simulink model "ZT_VehCtrl_18B"  (R2018b)
settings: Solver=FixedStepAuto  StartTime=0.0  StopTime=inf  FixedStep=0.005  RelTol=1e-3
InitFcn:
  | mbd_mpc_consistency_checks(bdroot(gcs));
undefined symbols (not defined in the file): ANG_DEAD, BMS_NormalPwr, BrkPrsByBrkPct_TB_X, BrkPrsByBrkPct_TB_Y, DELAY_DISCHARGE, DELAY_RCUOFF, DRV_BACKWARD, DRV_BRAKE, DRV_FORWARD, DRV_NEUTRAL, DRV_PARK, DRV_UNPARK, DRV_ZEROTURN, EPB_LOCK, EPB_UNLOCK, ExtraLoadPwr, FanOff, fifo_0_vect, fifo_1_vect, HiFanReq, HV_finished, HV_No_Active, HV_POWER_OFF, HV_POWER_ON, HVDown, HVON, KaTLS_v_DrgUp_X_VehSpd, KeFTM_s_Way1OffDlyTime, KeFTM_TK_Way1CoolLv2OffBatTemp, KeFTM_TK_Way1CoolLv2OffMtrTemp, KeFTM_TK_Way1CoolLv2OnBatTemp, KeFTM_TK_Way1CoolLv2OnMtrTemp, KeFTM_TK_Way1CoolLv3OffBatTemp, KeFTM_TK_Way1CoolLv3OffMtrTemp, KeFTM_TK_Way1CoolLv3OnBatTemp, KeFTM_TK_Way1CoolLv3OnMtrTemp, KeFTM_TK_Way1CoolLv4OffBatTemp, KeFTM_TK_Way1CoolLv4OffMtrTemp, KeFTM_TK_Way1CoolLv4OnBatTemp, KeFTM_TK_Way1CoolLv4OnMtrTemp, Kp1, Kp2, LowFanReq, LQFP, MtrPwrFactor_RCU, MtrPwrHighToMidThd, MtrPwrLowToMidThd, MtrPwrMidToHighThd, MtrPwrMidToLowThd, MtrTrqMax, PCT_DEAD, Precharge, PTO_1000, PTO_540, pts1_fifo_0_vect, pts1_fifo_1_vect, pts2_fifo_0_vect, pts2_fifo_1_vect, pts3_fifo_0_vect, pts3_fifo_1_vect ... (+24)
libraries: mbd_mpc574x_ec_toolbox x124, canmsglib x72, simulink x57
(part 10 of 11)

== system ZT_VehCtrl_18B/SigOut/GPIO /PWM_OUT/PWM Configuration and Frequency Update4 ==
  PWM A : Inport
  Fre : Inport  Port=2
  Add : Sum  Inputs=+-
  Constant : Constant
  Constant1 : Constant  Commented=on  Value=200
  Data Type Conversion : DataTypeConversion
  Data Type Conversion1 : DataTypeConversion  Commented=on
  FlexPWM_Config : mbd_mpc574x_ec_toolbox/Motor Control Blocks/FlexPWM Blocks/FlexPWM_Config  Priority=1  pwmModule=0  pwmSubmodule=1  pwmMode=Center aligned PWM  pwmPair=Independent  pwmCompSource=PWM23  pwmCounterInit=Local sync (PWMX)  pwmClockSource=Peripheral clock  pwmUnits=Hz  pwmFrequency=200  pwmPeriod=25000  pwmPrescaler=Divide by 16  pwmDtUnits=Nanoseconds  pwmDtNs=50  pwmDtTicks=4  pwmReloadLogic=Full Cycle  pwmReloadFrequency=Every 1 PWM opportunity  pwmTriggeringSignal=Local force signal  pwmDutyCycleOutSim=off  pwmStartAfterInit=on  pwmShowAdvOpts=off  pwmPinA=PTC7: [PWM0_A1 | FlexPWM_0 Channel A Input/Output 1]  pwmPinB=None  pwmPolarityA=off  pwmPolarityB=off  pwmAInitialVal=0.25  pwmBInitialVal=0.25  pwmAShift=0  pwmBShift=0  trgReloadISR=off  trgVal0=off  trgVal1=off  trgVal2=off  trgVal3=off  trgVal4=off  trgVal5=off  trgReloadErrorISR=off  pwmPinFault=None  PwmFaultEnISR=off  pwmFaultEnA=off  pwmFaultEnB=off
  FlexPWM_Frequency_Update : mbd_mpc574x_ec_toolbox/Motor Control Blocks/FlexPWM Blocks/FlexPWM_Frequency_Update  Priority=1  Commented=on  pwmModule=0  pwmSubmodule0=off  pwmSubmodule1=on  pwmSubmodule2=off  pwmSubmodule3=off  pwmUnits=Hz
  Terminator : Terminator
  wires:
  PWM A/1 -> Add/2
  Add/1 -> Data Type Conversion/1
  Constant/1 -> Add/1
  Data Type Conversion/1 -> FlexPWM_Config/1
  Fre/1 -> Terminator/1
  Constant1/1 -> Data Type Conversion1/1
  Data Type Conversion1/1 -> FlexPWM_Frequency_Update/1

== system ZT_VehCtrl_18B/SigOut/GPIO /SPI0: LS09_14_15_16_1_2_11_4/LS_CTRL ==
  Enable : EnablePort
  Data Type Conversion3 : DataTypeConversion
  Data Type Conversion4 : DataTypeConversion
  Demux1 : Demux  Outputs=2
  If Action Subsystem1 : Subsystem  TreatAsAtomicUnit=on
  SPI_Master_Transfer_To1 : mbd_mpc574x_ec_toolbox/Communication Blocks/SPI Blocks/SPI_Master_Transfer  Priority=2  InstanceNumber=0  xfermode=Non blocking  timeout=50  spi_upd=on  WhichPCS=5
  Terminator : Terminator
  Terminator1 : Terminator
  Vector Concatenate1 : Concatenate
  wires:
  Vector Concatenate1/1 -> SPI_Master_Transfer_To1/1
  SPI_Master_Transfer_To1/1 -> Demux1/1
  Demux1/2 -> Data Type Conversion4/1
  Data Type Conversion3/1 -> Terminator/1
  Data Type Conversion4/1 -> Terminator1/1
  Demux1/1 -> Data Type Conversion3/1
  If Action Subsystem1/1(Out1) -> Vector Concatenate1/1
  If Action Subsystem1/2(Out2) -> Vector Concatenate1/2

== system ZT_VehCtrl_18B/SigOut/GPIO /SPI0: LS09_14_15_16_1_2_11_4/LS_CTRL1 ==
  Enable : EnablePort
  Data Type Conversion3 : DataTypeConversion
  Data Type Conversion4 : DataTypeConversion
  Demux1 : Demux  Outputs=2
  If Action Subsystem1 : Subsystem  TreatAsAtomicUnit=on
  SPI_Master_Transfer_To1 : mbd_mpc574x_ec_toolbox/Communication Blocks/SPI Blocks/SPI_Master_Transfer  Priority=2  InstanceNumber=0  xfermode=Non blocking  timeout=50  spi_upd=on  WhichPCS=1
  Terminator : Terminator
  Terminator1 : Terminator
  Vector Concatenate1 : Concatenate
  wires:
  Demux1/1 -> Data Type Conversion3/1
  Data Type Conversion4/1 -> Terminator1/1
  Data Type Conversion3/1 -> Terminator/1
  Demux1/2 -> Data Type Conversion4/1
  SPI_Master_Transfer_To1/1 -> Demux1/1
  Vector Concatenate1/1 -> SPI_Master_Transfer_To1/1
  If Action Subsystem1/2(Out2) -> Vector Concatenate1/2
  If Action Subsystem1/1(Out1) -> Vector Concatenate1/1

== system ZT_VehCtrl_18B/SigOut/GPIO /SPI3: LS03_06_07_08_10_12_13_17_18_19/Subsystem ==
  Enable : EnablePort
  Data Type Conversion : DataTypeConversion  OutDataTypeStr=uint8
  Data Type Conversion1 : DataTypeConversion  OutDataTypeStr=uint8
  Demux2 : Demux  Outputs=2
  SPI_Master_Transfer_To2 : mbd_mpc574x_ec_toolbox/Communication Blocks/SPI Blocks/SPI_Master_Transfer  Priority=2  InstanceNumber=3  xfermode=Non blocking  timeout=50  spi_upd=on  WhichPCS=3
  Terminator2 : Terminator
  Terminator3 : Terminator
  Vector Concatenate2 : Concatenate
  控制 : Subsystem  TreatAsAtomicUnit=on
  wires:
  Data Type Conversion1/1 -> Terminator3/1
  控制/2(Out2) -> Vector Concatenate2/2
  Demux2/1 -> Data Type Conversion/1
  Vector Concatenate2/1 -> SPI_Master_Transfer_To2/1
  Demux2/2 -> Data Type Conversion1/1
  Data Type Conversion/1 -> Terminator2/1
  控制/1(Out1) -> Vector Concatenate2/1
  SPI_Master_Transfer_To2/1 -> Demux2/1

== system ZT_VehCtrl_18B/VehCtrl/MontionControl/DriveControl/Brake ==
  VehBrkTgt : Inport
  In2 : Inport  Port=2
  1-D Lookup Table : Lookup_n-D  NumberOfTableDimensions=1  BreakpointsForDimension1=BrkPrsByBrkPct_TB_X  Table=BrkPrsByBrkPct_TB_Y  InternalRulePriority=Speed  RndMeth=Simplest  InputSameDT=on
  Bus Selector : BusSelector  OutputSignals=NonDrive
  Constant : Constant
  Gain : Gain  Gain=0.01
  Switch : Switch  Criteria=u2 > Threshold
  BrkPrsTgt : Outport
  wires:
  VehBrkTgt/1 -> Gain/1  "VehBrkTgt"
  1-D Lookup Table/1 -> BrkPrsTgt/1
  Gain/1 -> Switch/3
  Switch/1 -> 1-D Lookup Table/1
  In2/1 -> Bus Selector/1
  Bus Selector/1 -> Switch/2  "<NonDrive>"
  Constant/1 -> Switch/1

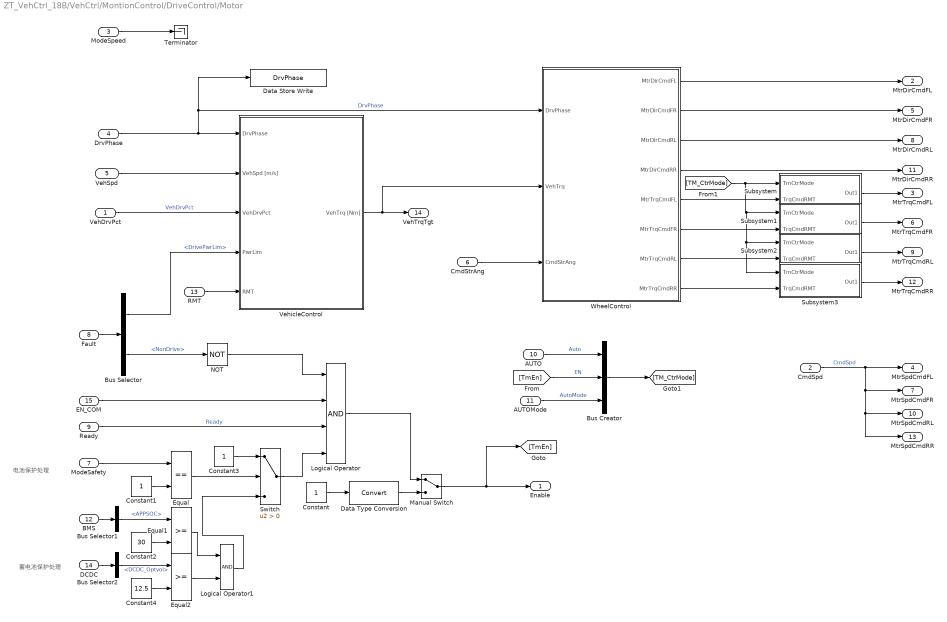
== system ZT_VehCtrl_18B/VehCtrl/MontionControl/DriveControl/Motor ==
  note: 电池保护处理
  note: 蓄电池保护处理
  VehDrvPct : Inport
  CmdSpd : Inport  Port=2
  ModeSpeed : Inport  Port=3
  DrvPhase : Inport  Port=4
  VehSpd : Inport  Port=5
  CmdStrAng : Inport  Port=6
  ModeSafety : Inport  Port=7
  Fault : Inport  Port=8
  Ready : Inport  Port=9
  AUTO : Inport  Port=10
  AUTOMode : Inport  Port=11
  BMS : Inport  Port=12
  RMT : Inport  Port=13
  DCDC : Inport  Port=14
  EN_COM : Inport  Port=15
  Bus Creator : BusCreator  Inputs=3
  Bus Selector : BusSelector  OutputSignals=DrivePwrLim,NonDrive
  Bus Selector1 : BusSelector  OutputSignals=BMS Power Infor.APPSOC
  Bus Selector2 : BusSelector  OutputSignals=DCDC_Optvol
  Constant : Constant
  Constant1 : Constant  OutDataTypeStr=boolean
  Constant2 : Constant  Value=30  OutDataTypeStr=boolean
  Constant3 : Constant  OutDataTypeStr=boolean
  Constant4 : Constant  Value=12.5  OutDataTypeStr=boolean
  Data Store Write : DataStoreWrite  DataStoreName=DrvPhase
  Data Type Conversion : DataTypeConversion
  Equal : RelationalOperator  Operator===  OutDataTypeStr=boolean  RndMeth=Simplest
  Equal1 : RelationalOperator  OutDataTypeStr=boolean  RndMeth=Simplest
  Equal2 : RelationalOperator  OutDataTypeStr=boolean  RndMeth=Simplest
  Logical Operator : Logic  Inputs=4  AllPortsSameDT=off  OutDataTypeStr=boolean
  Logical Operator1 : Logic  AllPortsSameDT=off  OutDataTypeStr=boolean
  Manual Switch : ManualSwitch
  NOT : Logic  Operator=NOT  IconShape=distinctive  AllPortsSameDT=off  OutDataTypeStr=boolean
  Subsystem : Subsystem
  Subsystem1 : Subsystem
  Subsystem2 : Subsystem
  Subsystem3 : Subsystem
  Switch : Switch  Criteria=u2 > Threshold
  Terminator : Terminator
  VehicleControl : Subsystem  TreatAsAtomicUnit=on
  WheelControl : Subsystem
  Enable : Outport
  MtrDirCmdFL : Outport  Port=2
  MtrTrqCmdFL : Outport  Port=3
  MtrSpdCmdFL : Outport  Port=4
  MtrDirCmdFR : Outport  Port=5
  MtrTrqCmdFR : Outport  Port=6
  MtrSpdCmdFR : Outport  Port=7
  MtrDirCmdRL : Outport  Port=8
  MtrTrqCmdRL : Outport  Port=9
  MtrSpdCmdRL : Outport  Port=10
  MtrDirCmdRR : Outport  Port=11
  MtrTrqCmdRR : Outport  Port=12
  MtrSpdCmdRR : Outport  Port=13
  VehTrqTgt : Outport  Port=14
  wires:
  VehSpd/1 -> VehicleControl/2(VehSpd [m/s])
  VehDrvPct/1 -> VehicleControl/3(VehDrvPct)  "VehDrvPct"
  DrvPhase/1 -> Data Store Write/1, WheelControl/1(DrvPhase), VehicleControl/1(DrvPhase)  "DrvPhase"
  CmdSpd/1 -> MtrSpdCmdRR/1, MtrSpdCmdRL/1, MtrSpdCmdFR/1, MtrSpdCmdFL/1  "CmdSpd"
  WheelControl/1(MtrDirCmdFL) -> MtrDirCmdFL/1
  WheelControl/2(MtrDirCmdFR) -> MtrDirCmdFR/1
  WheelControl/3(MtrDirCmdRL) -> MtrDirCmdRL/1
  WheelControl/4(MtrDirCmdRR) -> MtrDirCmdRR/1
  Fault/1 -> Bus Selector/1
  Bus Selector/1 -> VehicleControl/4(PwrLim)  "<DrivePwrLim>"
  Bus Selector/2 -> NOT/1  "<NonDrive>"
  NOT/1 -> Logical Operator/1
  Ready/1 -> Logical Operator/3  "Ready"
  Manual Switch/1 -> [TmEn], Enable/1
  VehicleControl/1(VehTrq [Nm]) -> WheelControl/2(VehTrq), VehTrqTgt/1
  CmdStrAng/1 -> WheelControl/3(CmdStrAng)
  WheelControl/5(MtrTrqCmdFL) -> Subsystem/2(TrqCmdRMT)
  WheelControl/6(MtrTrqCmdFR) -> Subsystem1/2(TrqCmdRMT)
  WheelControl/7(MtrTrqCmdRL) -> Subsystem2/2(TrqCmdRMT)
  WheelControl/8(MtrTrqCmdRR) -> Subsystem3/2(TrqCmdRMT)
  ModeSpeed/1 -> Terminator/1
  ModeSafety/1 -> Equal/1
  Constant1/1 -> Equal/2
  Equal/1 -> Switch/2
  Constant2/1 -> Equal1/2
  Logical Operator1/1 -> Switch/3
  Constant3/1 -> Switch/1
  Switch/1 -> Logical Operator/4
  AUTO/1 -> Bus Creator/1  "Auto"
  AUTOMode/1 -> Bus Creator/3  "AutoMode"
  BMS/1 -> Bus Selector1/1
  Bus Selector1/1 -> Equal1/1  "<APPSOC>"
  RMT/1 -> VehicleControl/5(RMT)
  Equal1/1 -> Logical Operator1/1
  Constant4/1 -> Equal2/2
  Equal2/1 -> Logical Operator1/2
  DCDC/1 -> Bus Selector2/1
  Bus Selector2/1 -> Equal2/1  "<DCDC_Optvol>"
  [TmEn] -> Bus Creator/2  "EN"
  Subsystem/1(Out1) -> MtrTrqCmdFL/1
  Bus Creator/1 -> [TM_CtrMode]
  [TM_CtrMode] -> Subsystem1/1(TmCtrMode), Subsystem3/1(TmCtrMode), Subsystem2/1(TmCtrMode), Subsystem/1(TmCtrMode)
  Subsystem1/1(Out1) -> MtrTrqCmdFR/1
  Subsystem2/1(Out1) -> MtrTrqCmdRL/1
  Subsystem3/1(Out1) -> MtrTrqCmdRR/1
  Constant/1 -> Data Type Conversion/1
  Data Type Conversion/1 -> Manual Switch/2
  Logical Operator/1 -> Manual Switch/1
  EN_COM/1 -> Logical Operator/2

== system ZT_VehCtrl_18B/VehCtrl/MontionControl/PtoControl/Subsystem ==
  ModeSpeed : Inport
  DirCmd : Inport  Port=2
  Add : Sum
  Constant : Constant  Value=16  OutDataTypeStr=uint8
  Constant1 : Constant  Value=4  OutDataTypeStr=uint8
  Constant2 : Constant  Value=32  OutDataTypeStr=uint8
  Constant3 : Constant  Value=0  OutDataTypeStr=uint8
  Switch : Switch  Criteria=u2 > Threshold
  Switch1 : Switch  Criteria=u2 > Threshold
  ModeReq : Outport
  wires:
  DirCmd/1 -> Switch/2
  Constant/1 -> Switch/1
  Constant1/1 -> Switch/3
  ModeSpeed/1 -> Switch1/2
  Constant2/1 -> Switch1/1
  Constant3/1 -> Switch1/3
  Switch1/1 -> Add/1
  Switch/1 -> Add/2
  Add/1 -> ModeReq/1

== system ZT_VehCtrl_18B/VehCtrl/MontionControl/PtoControl/Subsystem1 ==
  <RMT_PtoMode> : Inport
  Constant : Constant  Value=PTO_540
  Constant1 : Constant  Value=PTO_1000
  Constant2 : Constant  Value=540  OutDataTypeStr=single
  Constant3 : Constant  Value=1000  OutDataTypeStr=single
  Constant4 : Constant  Value=0  OutDataTypeStr=single
  Gain : Gain
  GreaterThan : RelationalOperator  Operator===  OutDataTypeStr=boolean  RndMeth=Simplest
  GreaterThan1 : RelationalOperator  Operator===  OutDataTypeStr=boolean  RndMeth=Simplest
  Switch : Switch  Criteria=u2 > Threshold
  Switch1 : Switch  Criteria=u2 > Threshold
  MtrSpdCmd : Outport
  wires:
  Switch1/1 -> Switch/3
  Constant4/1 -> Switch1/3
  Constant1/1 -> GreaterThan1/2
  GreaterThan1/1 -> Switch1/2
  Constant2/1 -> Switch/1
  Constant3/1 -> Switch1/1
  Constant/1 -> GreaterThan/2
  GreaterThan/1 -> Switch/2
  <RMT_PtoMode>/1 -> GreaterThan1/1, GreaterThan/1
  Switch/1 -> Gain/1
  Gain/1 -> MtrSpdCmd/1  "MtrSpdCmd"

== system ZT_VehCtrl_18B/VehCtrl/MontionControl/ValveControl/BrakeSys ==
  BrkPrsTgt : Inport
  BrkPrs : Inport  Port=2
  Chart : Stateflow chart  Commented=on  TreatAsAtomicUnit=on
  BrkValve : Outport
  wires:
  BrkPrs/1 -> Chart/1(BrkPrs)
  BrkPrsTgt/1 -> BrkValve/1, Chart/2(BrkPrsTgt)

== system ZT_VehCtrl_18B/VehCtrl/MontionControl/ValveControl/EpbSys ==
  EpbSt : Inport
  EpbValve : Outport
  wires:
  EpbSt/1 -> EpbValve/1

== system ZT_VehCtrl_18B/VehCtrl/MontionControl/ValveControl/PumpSys ==
  Ready : Inport
  Compare To Zero : simulink/Logic and Bit Operations/Compare To Zero  relop=>  OutDataTypeStr=boolean
  Pump : Outport
  wires:
  Compare To Zero/1 -> Pump/1
  Ready/1 -> Compare To Zero/1

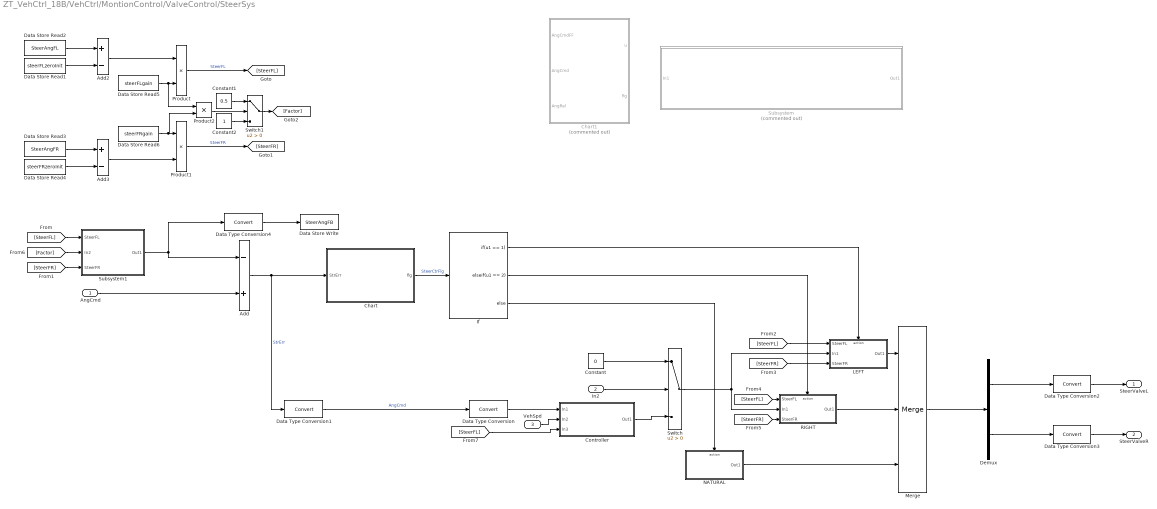
== system ZT_VehCtrl_18B/VehCtrl/MontionControl/ValveControl/SteerSys ==
  AngCmd : Inport
  In2 : Inport  Port=2
  VehSpd : Inport  Port=3
  Add : Sum  Inputs=-+
  Add2 : Sum  Inputs=+-
  Add3 : Sum  Inputs=+-
  Chart : Stateflow chart  TreatAsAtomicUnit=on
  Chart1 : Stateflow chart  Commented=on  TreatAsAtomicUnit=on
  Constant : Constant  Value=0  OutDataTypeStr=single
  Constant1 : Constant  Value=0.5  OutDataTypeStr=single
  Constant2 : Constant  OutDataTypeStr=single
  Controller : Subsystem
  Data Store Read1 : DataStoreRead  DataStoreName=steerFLzeroInit
  Data Store Read2 : DataStoreRead  DataStoreName=SteerAngFL
  Data Store Read3 : DataStoreRead  DataStoreName=SteerAngFR
  Data Store Read4 : DataStoreRead  DataStoreName=steerFRzeroInit
  Data Store Read5 : DataStoreRead  DataStoreName=steerFLgain
  Data Store Read6 : DataStoreRead  DataStoreName=steerFRgain
  Data Store Write : DataStoreWrite  DataStoreName=SteerAngFB
  Data Type Conversion{,1..4} (5 alike) : DataTypeConversion
  Demux : Demux  Outputs=2
  If : If  IfExpression=u1 == 1  ElseIfExpressions=u1 == 2
  LEFT : Subsystem  TreatAsAtomicUnit=on
  Merge : Merge  Inputs=3
  "NATURAL " : Subsystem  TreatAsAtomicUnit=on
  Product : Product
  Product1 : Product
  Product2 : Product
  RIGHT : Subsystem  TreatAsAtomicUnit=on
  Subsystem : Subsystem  Commented=on
  Subsystem1 : Subsystem
  Switch : Switch  Criteria=u2 > Threshold
  Switch1 : Switch  Criteria=u2 > Threshold
  SteerValveL : Outport
  SteerValveR : Outport  Port=2
  wires:
  If/1 -> LEFT/Action
  Switch/1 -> LEFT/2(In1), RIGHT/2(In1)
  If/2 -> RIGHT/Action
  If/3 -> "NATURAL "/Action
  RIGHT/1(Out1) -> Merge/2
  "NATURAL "/1(Out1) -> Merge/3
  LEFT/1(Out1) -> Merge/1
  Merge/1 -> Demux/1
  Data Type Conversion2/1 -> SteerValveL/1
  Data Type Conversion3/1 -> SteerValveR/1
  Demux/1 -> Data Type Conversion2/1
  Demux/2 -> Data Type Conversion3/1
  Subsystem1/1(Out1) -> Add/1, Data Type Conversion4/1
  Data Type Conversion4/1 -> Data Store Write/1
  Add/1 -> Chart/1(StrErr), Data Type Conversion1/1  "StrErr"
  Chart/1(flg) -> If/1  "SteerCtrFlg"
  Controller/1(Out1) -> Switch/3
  In2/1 -> Switch/2
  Constant/1 -> Switch/1
  AngCmd/1 -> Add/2
  VehSpd/1 -> Controller/2(In2)
  Data Type Conversion1/1 -> Data Type Conversion/1  "AngCmd"
  Add3/1 -> Product1/2
  Data Store Read4/1 -> Add3/2
  Data Store Read5/1 -> Product2/1, Product/2
  Data Store Read2/1 -> Add2/1
  Add2/1 -> Product/1
  Product1/1 -> [SteerFR]  "SteerFR"
  Data Store Read6/1 -> Product2/2, Product1/1
  Data Store Read1/1 -> Add2/2
  Data Store Read3/1 -> Add3/1
  Product/1 -> [SteerFL]  "SteerFL"
  [SteerFL] -> Subsystem1/1(SteerFL)
  [SteerFR] -> Subsystem1/3("SteerFR ")
  [SteerFR] -> LEFT/3(SteerFR)
  [SteerFL] -> LEFT/1("SteerFL ")
  [SteerFL] -> RIGHT/1(SteerFL)
  [SteerFR] -> RIGHT/3(SteerFR)
  Product2/1 -> Switch1/2
  Constant1/1 -> Switch1/1
  Constant2/1 -> Switch1/3
  Switch1/1 -> [Factor]
  [Factor] -> Subsystem1/2(In2)
  Data Type Conversion/1 -> Controller/1(In1)
  [SteerFL] -> Controller/3(In3)

== system ZT_VehCtrl_18B/VehCtrl/MontionControl/ValveControl/SuspesionSys ==
  note: 由于没有高度或长度传感器，初期为开环控制；
      | 后续考虑是否可以增加传感器，构建闭环控制。
  SuspSt : Inport
  ModeSafety : Inport  Port=2
  Constant{,1,3..4} (4 alike) : Constant  Value=false  OutDataTypeStr=boolean
  Constant2 : Constant  Value=true  OutDataTypeStr=boolean
  Constant5 : Constant  Value=true  OutDataTypeStr=boolean
  Constant6 : Constant  Value=0
  Data Type Conversion : DataTypeConversion
  Data Type Conversion1 : DataTypeConversion
  Data Type Conversion2 : DataTypeConversion  OutDataTypeStr=uint8
  Data Type Conversion3 : DataTypeConversion  OutDataTypeStr=uint8
  Data Type Conversion4 : DataTypeConversion  OutDataTypeStr=uint8
  Demux : Demux  Outputs=2
  Multiport Switch : MultiPortSwitch  DataPortOrder=Zero-based contiguous  zeroidx=on
  Mux : Mux  Inputs=2
  Mux1 : Mux  Inputs=2
  Mux2 : Mux  Inputs=2
  Switch1 : Switch  Criteria=u2 > Threshold
  SuspUpValve : Outport
  SuspDownValve : Outport  Port=2
  wires:
  Mux/1 -> Multiport Switch/2
  Mux1/1 -> Multiport Switch/3
  Mux2/1 -> Multiport Switch/4
  Constant/1 -> Mux/1
  Constant1/1 -> Mux/2
  Constant3/1 -> Mux1/2
  Constant2/1 -> Mux1/1
  Constant4/1 -> Mux2/1
  Constant5/1 -> Mux2/2
  Switch1/1 -> Data Type Conversion4/1
  Multiport Switch/1 -> Demux/1
  Demux/2 -> Data Type Conversion1/1
  Demux/1 -> Data Type Conversion/1
  Data Type Conversion/1 -> SuspUpValve/1
  Data Type Conversion1/1 -> SuspDownValve/1
  Data Type Conversion4/1 -> Multiport Switch/1  "suspmodeCtrl"
  ModeSafety/1 -> Switch1/2
  SuspSt/1 -> Data Type Conversion2/1
  Data Type Conversion2/1 -> Switch1/1
  Data Type Conversion3/1 -> Switch1/3
  Constant6/1 -> Data Type Conversion3/1

== system ZT_VehCtrl_18B/VehCtrl/MontionControl/ValveControl/WidthSys ==
  ModeSafety : Inport
  <RMT_ModeWidth> : Inport  Port=2
  Constant{,1,3..4} (4 alike) : Constant  Value=false  OutDataTypeStr=boolean
  Constant2 : Constant  Value=true  OutDataTypeStr=boolean
  Constant5 : Constant  Value=true  OutDataTypeStr=boolean
  Constant6 : Constant  Value=0  OutDataTypeStr=boolean
  Data Type Conversion : DataTypeConversion
  Data Type Conversion1 : DataTypeConversion
  Data Type Conversion2 : DataTypeConversion  OutDataTypeStr=uint8
  Data Type Conversion3 : DataTypeConversion  OutDataTypeStr=uint8
  Data Type Conversion4 : DataTypeConversion  OutDataTypeStr=uint8
  Demux : Demux  Outputs=2
  Multiport Switch : MultiPortSwitch  DataPortOrder=Zero-based contiguous  zeroidx=on
  Mux : Mux  Inputs=2
  Mux1 : Mux  Inputs=2
  Mux2 : Mux  Inputs=2
  Switch1 : Switch  Criteria=u2 > Threshold
  WidthLengthenValve : Outport
  WidthShortenValve : Outport  Port=2
  wires:
  Multiport Switch/1 -> Demux/1
  Demux/1 -> Data Type Conversion/1
  Demux/2 -> Data Type Conversion1/1
  Constant/1 -> Mux/1
  Mux2/1 -> Multiport Switch/4
  Constant2/1 -> Mux1/1
  Constant3/1 -> Mux1/2
  Mux1/1 -> Multiport Switch/3
  Mux/1 -> Multiport Switch/2
  Constant1/1 -> Mux/2
  Constant5/1 -> Mux2/2
  Constant4/1 -> Mux2/1
  Data Type Conversion/1 -> WidthLengthenValve/1
  Data Type Conversion1/1 -> WidthShortenValve/1
  ModeSafety/1 -> Switch1/2
  <RMT_ModeWidth>/1 -> Data Type Conversion2/1
  Constant6/1 -> Data Type Conversion3/1
  Switch1/1 -> Data Type Conversion4/1
  Data Type Conversion2/1 -> Switch1/1
  Data Type Conversion3/1 -> Switch1/3
  Data Type Conversion4/1 -> Multiport Switch/1  "widthmodeCtrl"

== system ZT_VehCtrl_18B/VehCtrl/TempertureControl/ThermFR_RRvRead1/Cnt_To_s ==
  In1 : Inport
  Constant1 : Constant  Value=200  OutDataTypeStr=uint8
  Data Type Conversion2 : DataTypeConversion  OutDataTypeStr=uint32
  Product1 : Product  OutDataTypeStr=fixdt(0,16,0.1,0)  RndMeth=Zero
  Out1 : Outport
  wires:
  Data Type Conversion2/1 -> Out1/1
  In1/1 -> Product1/1
  Product1/1 -> Data Type Conversion2/1
  Constant1/1 -> Product1/2

== system ZT_VehCtrl_18B/VehCtrl/TempertureControl/ThermFR_RRvRead2/Cnt_To_s ==
  In1 : Inport
  Constant1 : Constant  Value=200  OutDataTypeStr=uint8
  Data Type Conversion2 : DataTypeConversion  OutDataTypeStr=uint32
  Product1 : Product  OutDataTypeStr=fixdt(0,16,0.1,0)  RndMeth=Zero
  Out1 : Outport
  wires:
  Constant1/1 -> Product1/2
  Product1/1 -> Data Type Conversion2/1
  In1/1 -> Product1/1
  Data Type Conversion2/1 -> Out1/1

== system ZT_VehCtrl_18B/VehCtrl/TempertureControl/ThermLvRead3/Cnt_To_s ==
  In1 : Inport
  Constant1 : Constant  Value=200  OutDataTypeStr=uint8
  Data Type Conversion2 : DataTypeConversion  OutDataTypeStr=uint32
  Product1 : Product  OutDataTypeStr=fixdt(0,16,0.1,0)  RndMeth=Zero
  Out1 : Outport
  wires:
  Constant1/1 -> Product1/2
  Product1/1 -> Data Type Conversion2/1
  In1/1 -> Product1/1
  Data Type Conversion2/1 -> Out1/1

== system ZT_VehCtrl_18B/SigIn/PWM/Subsystem/eTimer Configuration and Signal Measurements/Subsystem_capture ==
  In1 : Inport
  function : TriggerPort  TriggerType=function-call  VariantControl=Variant
  Terminator : Terminator
  eTimer_Arm_Capture : mbd_mpc574x_ec_toolbox/Motor Control Blocks/eTIMER Blocks/eTimer_Arm_Capture  etimerModule=0  etimerChannel=1  etimerArmAction=Stop
  eTimer_Capture : mbd_mpc574x_ec_toolbox/Motor Control Blocks/eTIMER Blocks/eTimer_Capture  etimerModule=0  etimerChannel=1
  Out1 : Outport  OutDataTypeStr=uint16
  Out2 : Outport  Port=2  OutDataTypeStr=uint16
  Out3 : Outport  Port=3  OutDataTypeStr=uint16
  Out4 : Outport  Port=4  OutDataTypeStr=uint16
  wires:
  eTimer_Capture/1 -> Out1/1
  eTimer_Capture/4 -> Out4/1
  eTimer_Capture/3 -> Out3/1
  eTimer_Capture/2 -> Out2/1
  In1/1 -> Terminator/1

== system ZT_VehCtrl_18B/SigOut/GPIO /SPI0: LS09_14_15_16_1_2_11_4/LS_CTRL/If Action Subsystem1 ==
  Add : Sum  Inputs=++++
  Constant1 : Constant  Value=128  OutDataTypeStr=uint8
  Constant2 : Constant  Value=64  OutDataTypeStr=uint8
  Constant3 : Constant  Value=32  OutDataTypeStr=uint8
  Constant4 : Constant  Value=16  OutDataTypeStr=uint8
  Constant5 : Constant  Value=8  OutDataTypeStr=uint8
  Constant6 : Constant  Value=4  OutDataTypeStr=uint8
  Constant7 : Constant  Value=2  OutDataTypeStr=uint8
  Constant8 : Constant  OutDataTypeStr=uint8
  Constant9 : Constant  Value=128  OutDataTypeStr=uint8
  Data Store Read : DataStoreRead  DataStoreName=LS004
  Data Store Read4 : DataStoreRead  DataStoreName=LS011
  Data Store Read5 : DataStoreRead  DataStoreName=LS001
  Data Store Read6 : DataStoreRead  DataStoreName=LS002
  Data Type Conversion : DataTypeConversion
  Data Type Conversion1 : DataTypeConversion
  Switch{,1..3} (4 alike) : Switch  Criteria=u2 > Threshold
  Out1 : Outport
  Out2 : Outport  Port=2
  wires:
  Constant2/1 -> Switch/3
  Constant1/1 -> Switch/1
  Add/1 -> Data Type Conversion1/1
  Data Store Read6/1 -> Switch/2
  Constant7/1 -> Switch3/1
  Switch1/1 -> Add/2
  Constant5/1 -> Switch2/1
  Switch/1 -> Add/1
  Constant4/1 -> Switch1/3
  Data Store Read/1 -> Switch3/2
  Switch2/1 -> Add/3
  Data Store Read4/1 -> Switch2/2
  Switch3/1 -> Add/4
  Constant3/1 -> Switch1/1
  Data Store Read5/1 -> Switch1/2
  Constant8/1 -> Switch3/3
  Constant9/1 -> Data Type Conversion/1
  Constant6/1 -> Switch2/3
  Data Type Conversion/1 -> Out1/1
  Data Type Conversion1/1 -> Out2/1

== system ZT_VehCtrl_18B/SigOut/GPIO /SPI0: LS09_14_15_16_1_2_11_4/LS_CTRL1/If Action Subsystem1 ==
  Add : Sum  Inputs=++++
  Constant1 : Constant  Value=128  OutDataTypeStr=uint8
  Constant2 : Constant  Value=64  OutDataTypeStr=uint8
  Constant3 : Constant  Value=32  OutDataTypeStr=uint8
  Constant4 : Constant  Value=16  OutDataTypeStr=uint8
  Constant5 : Constant  Value=8  OutDataTypeStr=uint8
  Constant6 : Constant  Value=4  OutDataTypeStr=uint8
  Constant7 : Constant  Value=2  OutDataTypeStr=uint8
  Constant8 : Constant  OutDataTypeStr=uint8
  Constant9 : Constant  Value=128  OutDataTypeStr=uint8
  Data Store Read : DataStoreRead  DataStoreName=LS014
  Data Store Read4 : DataStoreRead  DataStoreName=LS015
  Data Store Read5 : DataStoreRead  DataStoreName=LS009
  Data Store Read6 : DataStoreRead  DataStoreName=LS016
  Data Type Conversion : DataTypeConversion
  Data Type Conversion1 : DataTypeConversion
  Switch{,1..3} (4 alike) : Switch  Criteria=u2 > Threshold
  Out1 : Outport
  Out2 : Outport  Port=2
  wires:
  Data Type Conversion1/1 -> Out2/1
  Data Type Conversion/1 -> Out1/1
  Constant6/1 -> Switch2/3
  Constant9/1 -> Data Type Conversion/1
  Constant8/1 -> Switch3/3
  Data Store Read5/1 -> Switch1/2
  Constant3/1 -> Switch1/1
  Switch3/1 -> Add/4
  Data Store Read4/1 -> Switch2/2
  Switch2/1 -> Add/3
  Data Store Read/1 -> Switch3/2
  Constant4/1 -> Switch1/3
  Switch/1 -> Add/1
  Constant5/1 -> Switch2/1
  Switch1/1 -> Add/2
  Constant7/1 -> Switch3/1
  Data Store Read6/1 -> Switch/2
  Add/1 -> Data Type Conversion1/1
  Constant1/1 -> Switch/1
  Constant2/1 -> Switch/3

== system ZT_VehCtrl_18B/SigOut/GPIO /SPI3: LS03_06_07_08_10_12_13_17_18_19/Subsystem/控制 ==
  note: out1
  note: out2
  note: out3
  note: out5
  note: out4
  note: out7
  note: out6
  note: out8
  Add : Sum  Inputs=++++++++
  Add1 : Sum  Inputs=+++
  Constant1 : Constant  Value=0
  Constant2 : Constant  Value=0
  Constant9 : Constant  Value=44  OutDataTypeStr=uint8
  Data Store Read : DataStoreRead  DataStoreName=LS019
  Data Store Read1 : DataStoreRead  DataStoreName=LS007
  Data Store Read10 : DataStoreRead  DataStoreName=LS006
  Data Store Read2 : DataStoreRead  DataStoreName=LS012
  Data Store Read4 : DataStoreRead  DataStoreName=LS018
  Data Store Read5 : DataStoreRead  DataStoreName=LS010
  Data Store Read6 : DataStoreRead  DataStoreName=LS008
  Data Store Read7 : DataStoreRead  DataStoreName=LS003
  Data Store Read8 : DataStoreRead  DataStoreName=LS017
  Data Store Read9 : DataStoreRead  DataStoreName=LS013
  Data Type Conversion : DataTypeConversion  OutDataTypeStr=uint8
  Data Type Conversion1 : DataTypeConversion  OutDataTypeStr=uint8
  Gain : Gain
  Gain1 : Gain  Gain=2
  Gain2 : Gain  Gain=4
  Gain3 : Gain  Gain=8
  Gain4 : Gain  Gain=16
  Gain5 : Gain  Gain=32
  Gain6 : Gain  Gain=64
  Gain7 : Gain  Gain=128
  Gain8 : Gain
  Gain9 : Gain  Gain=2
  Terminator{,1..3} (4 alike) : Terminator
  Out1 : Outport  VectorParamsAs1DForOutWhenUnconnected=on
  Out2 : Outport  Port=2  VectorParamsAs1DForOutWhenUnconnected=on
  wires:
  Constant9/1 -> Add1/1
  Data Store Read10/1 -> Gain7/1
  Data Type Conversion1/1 -> Out2/1
  Data Store Read2/1 -> Gain9/1
  Add1/1 -> Data Type Conversion/1
  Add/1 -> Data Type Conversion1/1
  Data Store Read5/1 -> Gain2/1
  Gain6/1 -> Add/2
  Data Store Read1/1 -> Gain8/1
  Gain9/1 -> Add1/2
  Gain7/1 -> Add/1
  Gain/1 -> Add/8
  Data Type Conversion/1 -> Out1/1
  Data Store Read9/1 -> Gain6/1
  Gain4/1 -> Add/4
  Gain8/1 -> Add1/3
  Gain1/1 -> Add/7
  Data Store Read6/1 -> Gain3/1
  Gain3/1 -> Add/5
  Gain2/1 -> Add/6
  Gain5/1 -> Add/3
  Data Store Read8/1 -> Terminator/1
  Data Store Read7/1 -> Terminator1/1
  Constant1/1 -> Gain4/1, Gain5/1
  Data Store Read/1 -> Terminator3/1
  Data Store Read4/1 -> Terminator2/1
  Constant2/1 -> Gain/1, Gain1/1

== system ZT_VehCtrl_18B/VehCtrl/MontionControl/DriveControl/Motor/Subsystem ==
  TmCtrMode : Inport
  TrqCmdRMT : Inport  Port=2
  Bus Selector3 : BusSelector  OutputSignals=Auto.signal3.AUTO_TrqCmdFL,EN,AutoMode
  Compare To Constant : simulink/Logic and Bit Operations/Compare To Constant  relop===  const=1  OutDataTypeStr=boolean
  Constant : Constant  Value=0
  Data Store Read : DataStoreRead  DataStoreName=CtrMode
  Data Type Conversion : DataTypeConversion
  Switch1 : Switch  Criteria=u2 > Threshold
  Switch3 : Switch  Criteria=u2 > Threshold
  Terminator : Terminator
  Out1 : Outport
  wires:
  Switch3/1 -> Out1/1
  TmCtrMode/1 -> Bus Selector3/1
  Bus Selector3/1 -> [TrqCmd]  "<AUTO_TrqCmdFL>"
  Bus Selector3/2 -> [EN]  "<EN>"
  Bus Selector3/3 -> [AutoMode]  "<AutoMode>"
  TrqCmdRMT/1 -> Switch1/3  "TrqCmdFL_RMT"
  [TrqCmd] -> Switch1/1  "TrqCmdFL_Auto"
  [EN] -> Switch3/2
  Constant/1 -> Data Type Conversion/1
  Switch1/1 -> Switch3/1  "TrqCtrFL"
  Compare To Constant/1 -> Switch1/2
  Data Store Read/1 -> Compare To Constant/1
  [AutoMode] -> Terminator/1
  Data Type Conversion/1 -> Switch3/3

== system ZT_VehCtrl_18B/VehCtrl/MontionControl/DriveControl/Motor/Subsystem1 ==
  TmCtrMode : Inport
  TrqCmdRMT : Inport  Port=2
  Bus Selector3 : BusSelector  OutputSignals=Auto.signal3.AUTO_TrqCmdFR,EN,AutoMode
  Compare To Constant : simulink/Logic and Bit Operations/Compare To Constant  relop===  const=1  OutDataTypeStr=boolean
  Constant : Constant  Value=0
  Data Store Read : DataStoreRead  DataStoreName=CtrMode
  Data Type Conversion : DataTypeConversion
  Switch1 : Switch  Criteria=u2 > Threshold
  Switch3 : Switch  Criteria=u2 > Threshold
  Terminator : Terminator
  Out1 : Outport
  wires:
  Switch1/1 -> Switch3/1
  Constant/1 -> Data Type Conversion/1
  [EN] -> Switch3/2
  [TrqCmd] -> Switch1/1
  TrqCmdRMT/1 -> Switch1/3
  Compare To Constant/1 -> Switch1/2
  Bus Selector3/3 -> [AutoMode]  "<AutoMode>"
  Bus Selector3/2 -> [EN]  "<EN>"
  Bus Selector3/1 -> [TrqCmd]  "<AUTO_TrqCmdFR>"
  TmCtrMode/1 -> Bus Selector3/1
  Switch3/1 -> Out1/1
  Data Store Read/1 -> Compare To Constant/1
  [AutoMode] -> Terminator/1
  Data Type Conversion/1 -> Switch3/3

== system ZT_VehCtrl_18B/VehCtrl/MontionControl/DriveControl/Motor/Subsystem2 ==
  TmCtrMode : Inport
  TrqCmdRMT : Inport  Port=2
  Bus Selector3 : BusSelector  OutputSignals=Auto.signal3.AUTO_TrqCmdRL,EN,AutoMode
  Compare To Constant : simulink/Logic and Bit Operations/Compare To Constant  relop===  const=1  OutDataTypeStr=boolean
  Constant : Constant  Value=0
  Data Store Read : DataStoreRead  DataStoreName=CtrMode
  Data Type Conversion : DataTypeConversion
  Switch1 : Switch  Criteria=u2 > Threshold
  Switch3 : Switch  Criteria=u2 > Threshold
  Terminator : Terminator
  Out1 : Outport
  wires:
  Switch3/1 -> Out1/1
  TmCtrMode/1 -> Bus Selector3/1
  Bus Selector3/1 -> [TrqCmd]  "<AUTO_TrqCmdRL>"
  Bus Selector3/2 -> [EN]  "<EN>"
  Bus Selector3/3 -> [AutoMode]  "<AutoMode>"
  Compare To Constant/1 -> Switch1/2
  TrqCmdRMT/1 -> Switch1/3
  [TrqCmd] -> Switch1/1
  [EN] -> Switch3/2
  Constant/1 -> Data Type Conversion/1
  Switch1/1 -> Switch3/1
  Data Store Read/1 -> Compare To Constant/1
  [AutoMode] -> Terminator/1
  Data Type Conversion/1 -> Switch3/3

== system ZT_VehCtrl_18B/VehCtrl/MontionControl/DriveControl/Motor/Subsystem3 ==
  TmCtrMode : Inport
  TrqCmdRMT : Inport  Port=2
  Bus Selector3 : BusSelector  OutputSignals=Auto.signal3.AUTO_TrqCmdRR,EN,AutoMode
  Compare To Constant : simulink/Logic and Bit Operations/Compare To Constant  relop===  const=1  OutDataTypeStr=boolean
  Constant : Constant  Value=0
  Data Store Read : DataStoreRead  DataStoreName=CtrMode
  Data Type Conversion : DataTypeConversion
  Switch1 : Switch  Criteria=u2 > Threshold
  Switch3 : Switch  Criteria=u2 > Threshold
  Terminator : Terminator
  Out1 : Outport
  wires:
  Switch1/1 -> Switch3/1
  Constant/1 -> Data Type Conversion/1
  [EN] -> Switch3/2
  [TrqCmd] -> Switch1/1
  TrqCmdRMT/1 -> Switch1/3
  Compare To Constant/1 -> Switch1/2
  Bus Selector3/3 -> [AutoMode]  "<AutoMode>"
  Bus Selector3/2 -> [EN]  "<EN>"
  Bus Selector3/1 -> [TrqCmd]  "<AUTO_TrqCmdRR>"
  TmCtrMode/1 -> Bus Selector3/1
  Switch3/1 -> Out1/1
  Data Store Read/1 -> Compare To Constant/1
  [AutoMode] -> Terminator/1
  Data Type Conversion/1 -> Switch3/3

== system ZT_VehCtrl_18B/VehCtrl/MontionControl/DriveControl/Motor/VehicleControl ==
  DrvPhase : Inport
  VehSpd [m/s] : Inport  Port=2
  VehDrvPct : Inport  Port=3
  PwrLim : Inport  Port=4
  RMT : Inport  Port=5
  Bus Selector1 : BusSelector  OutputSignals=RMT2.RMT_MtrTqGr
  Constant1 : Constant  Value=DRV_BACKWARD
  Constant2 : Constant  Value=DRV_FORWARD
  Constant3 : Constant  Value=0.0  OutDataTypeStr=single
  GreaterThan1 : RelationalOperator  Operator===  OutDataTypeStr=boolean  RndMeth=Simplest
  GreaterThan2 : RelationalOperator  Operator===  OutDataTypeStr=boolean  RndMeth=Simplest
  Product : Product
  Switch1 : Switch  Criteria=u2 > Threshold
  Switch2 : Switch  Criteria=u2 > Threshold
  VehTrqBackward : Subsystem
  VehTrqForward : Subsystem
  VehTrq [Nm] : Outport
  wires:
  DrvPhase/1 -> GreaterThan2/1, GreaterThan1/1
  Switch1/1 -> Product/1  "VehTrq"
  Constant1/1 -> GreaterThan1/2
  GreaterThan1/1 -> Switch1/2
  Switch2/1 -> Switch1/3
  Constant2/1 -> GreaterThan2/2
  GreaterThan2/1 -> Switch2/2
  VehTrqBackward/1(VehTrq) -> Switch1/1
  VehTrqForward/1(VehTrq) -> Switch2/1
  Constant3/1 -> Switch2/3
  VehDrvPct/1 -> VehTrqForward/2(VehDrv), VehTrqBackward/2(VehDrvPct)
  VehSpd [m/s]/1 -> VehTrqForward/1(VehSpd), VehTrqBackward/1(VehSpd)
  PwrLim/1 -> VehTrqForward/3(PwrLim), VehTrqBackward/3(PwrLim)
  RMT/1 -> Bus Selector1/1
  Bus Selector1/1 -> Product/2  "<RMT_MtrTqGr>"
  Product/1 -> VehTrq [Nm]/1  "VehTrq_ter"

== system ZT_VehCtrl_18B/VehCtrl/MontionControl/DriveControl/Motor/WheelControl ==
  DrvPhase : Inport
  VehTrq : Inport  Port=2
  CmdStrAng : Inport  Port=3
  Chart : Stateflow chart  TreatAsAtomicUnit=on
  Constant : Constant  Value=MtrTrqMax
  Data Store Read : DataStoreRead  DataStoreName=MtrTrqZeroturn
  Data Store Read1 : DataStoreRead  DataStoreName=FacFrontInter
  Data Store Read2 : DataStoreRead  DataStoreName=FacFrontOuter
  Data Store Read3 : DataStoreRead  DataStoreName=FacRearInter
  Data Store Read4 : DataStoreRead  DataStoreName=FacRearOuter
  MtrDirCmdFL : Outport
  MtrDirCmdFR : Outport  Port=2
  MtrDirCmdRL : Outport  Port=3
  MtrDirCmdRR : Outport  Port=4
  MtrTrqCmdFL : Outport  Port=5
  MtrTrqCmdFR : Outport  Port=6
  MtrTrqCmdRL : Outport  Port=7
  MtrTrqCmdRR : Outport  Port=8
  wires:
  Chart/5(MtrTrqCmdFL) -> MtrTrqCmdFL/1
  Chart/4(MtrDirCmdRR) -> MtrDirCmdRR/1  "MtrDirCmdRR"
  VehTrq/1 -> Chart/2(VehTrq)
  Chart/2(MtrDirCmdFR) -> MtrDirCmdFR/1  "MtrDirCmdFR"
  Chart/8(MtrTrqCmdRR) -> MtrTrqCmdRR/1
  Chart/6(MtrTrqCmdFR) -> MtrTrqCmdFR/1
  Chart/7(MtrTrqCmdRL) -> MtrTrqCmdRL/1
  Chart/1(MtrDirCmdFL) -> MtrDirCmdFL/1  "MtrDirCmdFL"
  CmdStrAng/1 -> Chart/4(CmdStrAng)
  Chart/3(MtrDirCmdRL) -> MtrDirCmdRL/1  "MtrDirCmdRL"
  DrvPhase/1 -> Chart/1(DrvPhase)
  Data Store Read/1 -> Chart/5(MtrTrqZeroturn)
  Data Store Read1/1 -> Chart/6(FacFrontInter)
  Data Store Read2/1 -> Chart/7(FacFrontOuter)
  Data Store Read4/1 -> Chart/9(FacRearOuter)
  Data Store Read3/1 -> Chart/8(FacRearInter)
  Constant/1 -> Chart/3(TrqMax)

== system ZT_VehCtrl_18B/VehCtrl/MontionControl/ValveControl/SteerSys/Controller ==
  In1 : Inport
  In2 : Inport  Port=2
  In3 : Inport  Port=3
  1-D Lookup Table : Lookup_n-D  NumberOfTableDimensions=1  BreakpointsForDimension1=VehSpd  Table=Kp1  InternalRulePriority=Speed  RndMeth=Simplest  InputSameDT=on
  1-D Lookup Table1 : Lookup_n-D  NumberOfTableDimensions=1  BreakpointsForDimension1=VehSpd  Table=Kp2  InternalRulePriority=Speed  RndMeth=Simplest  InputSameDT=on
  Abs : Abs
  Add : Sum
  Data Store Read : DataStoreRead  DataStoreName=Kd
  Data Type Conversion : DataTypeConversion  OutDataTypeStr=double
  Data Type Conversion1 : DataTypeConversion  OutDataTypeStr=single
  Data Type Conversion2 : DataTypeConversion  OutDataTypeStr=double
  Dead Zone : DeadZone  LowerValue=-15  UpperValue=15  SaturateOnIntegerOverflow=on
  Derivative2 : Derivative
  Product : Product
  Product1 : Product
  Saturation : Saturate  UpperLimit=100  LowerLimit=-100
  Saturation1 : Saturate  UpperLimit=36  LowerLimit=18
  Switch : Switch  Criteria=u2 > Threshold
  Out1 : Outport
  wires:
  Data Type Conversion1/1 -> Saturation/1
  Saturation/1 -> Dead Zone/1
  Saturation1/1 -> Product/2  "kp"
  In1/1 -> Data Type Conversion/1
  Abs/1 -> Out1/1
  Dead Zone/1 -> Abs/1
  In2/1 -> Data Type Conversion2/1
  Data Type Conversion2/1 -> 1-D Lookup Table1/1, 1-D Lookup Table/1
  1-D Lookup Table/1 -> Switch/1
  Data Type Conversion/1 -> Product1/2, Product/1
  Derivative2/1 -> Add/1
  Product1/1 -> Derivative2/1
  Data Store Read/1 -> Product1/1
  Add/1 -> Data Type Conversion1/1
  Product/1 -> Add/2
  In3/1 -> Switch/2
  1-D Lookup Table1/1 -> Switch/3
  Switch/1 -> Saturation1/1

== system ZT_VehCtrl_18B/VehCtrl/MontionControl/ValveControl/SteerSys/LEFT ==
  note: 左正右负，左转限制左边幅值
  "SteerFL " : Inport
  In1 : Inport  Port=2
  SteerFR : Inport  Port=3
  Action Port : ActionPort  ActionType=then
  Add1 : Sum  Inputs=-+
  Add4 : Sum  Inputs=-+
  Compare To Constant : simulink/Logic and Bit Operations/Compare To Constant  relop=>  const=0  OutDataTypeStr=boolean
  Compare To Constant1 : simulink/Logic and Bit Operations/Compare To Constant  relop=>  const=0  OutDataTypeStr=boolean
  Constant : Constant  Value=0  OutDataTypeStr=single
  Constant1 : Constant  Value=SteerAngMax
  Constant2 : Constant
  Constant3 : Constant  Value=0
  Constant6 : Constant  Value=SteerAngMax
  Data Type Conversion : DataTypeConversion
  Logical Operator : Logic  Operator=OR  AllPortsSameDT=off  OutDataTypeStr=boolean
  Mux : Mux  Inputs=2
  Product2 : Product
  Switch1 : Switch  Criteria=u2 > Threshold
  Out1 : Outport
  wires:
  Constant/1 -> Mux/2
  In1/1 -> Product2/2
  Mux/1 -> Out1/1
  Constant2/1 -> Switch1/3
  Constant3/1 -> Switch1/1
  Constant1/1 -> Add1/1
  Switch1/1 -> [SteerK]
  [SteerK] -> Product2/1
  Product2/1 -> Data Type Conversion/1
  Data Type Conversion/1 -> Mux/1
  Constant6/1 -> Add4/1
  Add1/1 -> Compare To Constant/1
  Add4/1 -> Compare To Constant1/1
  Logical Operator/1 -> Switch1/2
  Compare To Constant/1 -> Logical Operator/1
  Compare To Constant1/1 -> Logical Operator/2
  "SteerFL "/1 -> Add1/2
  SteerFR/1 -> Add4/2

== system ZT_VehCtrl_18B/VehCtrl/MontionControl/ValveControl/SteerSys/NATURAL  ==
  Action Port : ActionPort  ActionType=else
  Constant : Constant  Value=0  OutDataTypeStr=single
  Constant1 : Constant  Value=0  OutDataTypeStr=single
  Mux : Mux  Inputs=2
  Out1 : Outport
  wires:
  Constant/1 -> Mux/1
  Mux/1 -> Out1/1
  Constant1/1 -> Mux/2

== system ZT_VehCtrl_18B/VehCtrl/MontionControl/ValveControl/SteerSys/RIGHT ==
  note: 左正右负，右转限制右边幅值
  SteerFL : Inport
  In1 : Inport  Port=2
  SteerFR : Inport  Port=3
  Action Port : ActionPort  ActionType=elseif
  Add3 : Sum  Inputs=-+
  Add6 : Sum  Inputs=-+
  Compare To Constant : simulink/Logic and Bit Operations/Compare To Constant  relop=>  const=0  OutDataTypeStr=boolean
  Compare To Constant1 : simulink/Logic and Bit Operations/Compare To Constant  relop=>  const=0  OutDataTypeStr=boolean
  Constant1 : Constant
  Constant2 : Constant  Value=0
  Constant4 : Constant  Value=0  OutDataTypeStr=single
  Constant5 : Constant  Value=SteerAngMax
  Constant8 : Constant  Value=SteerAngMax
  Data Type Conversion : DataTypeConversion
  Gain : Gain  Gain=-1
  Gain1 : Gain  Gain=-1
  Logical Operator : Logic  Operator=OR  AllPortsSameDT=off  OutDataTypeStr=boolean
  Mux : Mux  Inputs=2
  Product1 : Product
  Switch1 : Switch  Criteria=u2 > Threshold
  Out1 : Outport
  wires:
  Mux/1 -> Out1/1
  Constant4/1 -> Mux/1
  Constant1/1 -> Switch1/3
  Constant2/1 -> Switch1/1
  Switch1/1 -> [SteerK]
  Logical Operator/1 -> Switch1/2
  [SteerK] -> Product1/2
  In1/1 -> Product1/1
  Product1/1 -> Data Type Conversion/1
  Data Type Conversion/1 -> Mux/2
  Constant5/1 -> Add3/1
  Compare To Constant1/1 -> Logical Operator/2
  Compare To Constant/1 -> Logical Operator/1
  Add6/1 -> Compare To Constant1/1
  Constant8/1 -> Add6/1
  Add3/1 -> Compare To Constant/1
  Gain/1 -> Add3/2
  Gain1/1 -> Add6/2
  SteerFL/1 -> Gain/1
  SteerFR/1 -> Gain1/1

== system ZT_VehCtrl_18B/VehCtrl/MontionControl/ValveControl/SteerSys/Subsystem ==
  In1 : Inport
  Abs1 : Abs
  If1 : If  ElseIfExpressions=u1 < 0
  LEFT1 : Subsystem  TreatAsAtomicUnit=on
  Merge1 : Merge  Inputs=3
  NATURAL 1 : Subsystem  TreatAsAtomicUnit=on
  RIGHT1 : Subsystem  TreatAsAtomicUnit=on
  Out1 : Outport
  wires:
  LEFT1/1(Out1) -> Merge1/1
  In1/1 -> If1/1, Abs1/1
  Abs1/1 -> RIGHT1/1(In1), LEFT1/1(In1)
  NATURAL 1/1(Out1) -> Merge1/3
  If1/3 -> NATURAL 1/Action
  If1/2 -> RIGHT1/Action
  RIGHT1/1(Out1) -> Merge1/2
  If1/1 -> LEFT1/Action
  Merge1/1 -> Out1/1

== system ZT_VehCtrl_18B/VehCtrl/MontionControl/ValveControl/SteerSys/Subsystem1 ==
  SteerFL : Inport
  In2 : Inport  Port=2
  "SteerFR " : Inport  Port=3
  Add : Sum
  Product : Product
  Out1 : Outport
  wires:
  Add/1 -> Product/1
  Product/1 -> Out1/1
  SteerFL/1 -> Add/1
  "SteerFR "/1 -> Add/2
  In2/1 -> Product/2

== system ZT_VehCtrl_18B/VehCtrl/MontionControl/DriveControl/Motor/VehicleControl/VehTrqBackward ==
  VehSpd : Inport
  VehDrvPct : Inport  Port=2
  PwrLim : Inport  Port=3
  Abs : Abs
  Constant : Constant  Value=VehTrqBackwardMax
  Constant1 : Constant  Value=VehPwrBackwardMax
  Constant2 : Constant  Value=WhlRadius
  Constant3 : Constant  Value=0.1  OutDataTypeStr=single
  Divide : Product  Inputs=*/
  Divide1 : Product  Inputs=*/
  Gain : Gain  Gain=1000
  Gain1 : Gain  Gain=0.01
  Gain2 : Gain  Gain=PwrLimFactor
  Max : MinMax  Function=max  Inputs=2
  Min : MinMax  Inputs=2
  Product : Product
  Product1 : Product
  Product2 : Product
  Switch : Switch  Criteria=u2 > Threshold
  VehTrq : Outport
  wires:
  VehDrvPct/1 -> Gain1/1
  Constant/1 -> Product1/2
  Product1/1 -> Min/1
  Gain1/1 -> Product/2, Product/1, Product1/1
  Product2/1 -> Divide/1
  Divide1/1 -> Divide/2
  Product/1 -> Product2/1
  Divide/1 -> Min/2
  Min/1 -> VehTrq/1
  Constant2/1 -> Divide1/2
  Constant3/1 -> Max/2
  Max/1 -> Divide1/1
  VehSpd/1 -> Abs/1
  Abs/1 -> Max/1
  Switch/1 -> Product2/2
  Constant1/1 -> Gain/1
  PwrLim/1 -> Switch/2
  Gain2/1 -> Switch/1
  Gain/1 -> Switch/3, Gain2/1

== system ZT_VehCtrl_18B/VehCtrl/MontionControl/DriveControl/Motor/VehicleControl/VehTrqForward ==
  VehSpd : Inport
  VehDrv : Inport  Port=2
  PwrLim : Inport  Port=3
  Abs : Abs
  Constant : Constant  Value=VehTrqMax
  Constant1 : Constant  Value=VehPwrMax
  Constant2 : Constant  Value=WhlRadius
  Constant3 : Constant  Value=0.1  OutDataTypeStr=single
  Divide : Product  Inputs=*/
  Divide1 : Product  Inputs=*/
  Gain : Gain  Gain=1000
  Gain1 : Gain  Gain=0.01
  Gain2 : Gain  Gain=PwrLimFactor
  Max : MinMax  Function=max  Inputs=2
  Min : MinMax  Inputs=2
  Product : Product
  Product1 : Product
  Product2 : Product
  Switch : Switch  Criteria=u2 > Threshold
  VehTrq : Outport
  wires:
  Gain2/1 -> Switch/1
  PwrLim/1 -> Switch/2
  Constant1/1 -> Gain/1
  Switch/1 -> Product2/2
  Abs/1 -> Max/1
  VehSpd/1 -> Abs/1
  Max/1 -> Divide1/1
  Constant3/1 -> Max/2
  Constant2/1 -> Divide1/2
  Min/1 -> VehTrq/1
  Divide/1 -> Min/2
  Product/1 -> Product2/1
  Divide1/1 -> Divide/2
  Product2/1 -> Divide/1
  Gain1/1 -> Product/1, Product/2, Product1/1
  Product1/1 -> Min/1
  VehDrv/1 -> Gain1/1
  Gain/1 -> Gain2/1, Switch/3
  Constant/1 -> Product1/2

== system ZT_VehCtrl_18B/VehCtrl/MontionControl/ValveControl/SteerSys/Subsystem/LEFT1 ==
  note: 左正右负，左转限制左边幅值
  In1 : Inport
  Action Port : ActionPort
  Add1 : Sum  Inputs=-+
  Add2 : Sum  Inputs=+-
  Add3 : Sum  Inputs=+-
  Add4 : Sum  Inputs=-+
  Compare To Constant : simulink/Logic and Bit Operations/Compare To Constant  relop=>  const=0  OutDataTypeStr=boolean
  Compare To Constant1 : simulink/Logic and Bit Operations/Compare To Constant  relop=>  const=0  OutDataTypeStr=boolean
  Constant : Constant  Value=0  OutDataTypeStr=single
  Constant1 : Constant  Value=SteerAngMax
  Constant2 : Constant
  Constant3 : Constant  Value=0
  Constant4 : Constant  Value=steerFLzeroInit
  Constant5 : Constant  Value=steerFRzeroInit
  Constant6 : Constant  Value=SteerAngMax
  Data Store Read2 : DataStoreRead  DataStoreName=SteerAngFL
  Data Store Read3 : DataStoreRead  DataStoreName=SteerAngFR
  Data Type Conversion : DataTypeConversion
  Logical Operator : Logic  Operator=OR  AllPortsSameDT=off  OutDataTypeStr=boolean
  Mux : Mux  Inputs=2
  Product2 : Product
  Switch1 : Switch  Criteria=u2 > Threshold
  Out1 : Outport
  wires:
  Compare To Constant1/1 -> Logical Operator/2
  Compare To Constant/1 -> Logical Operator/1
  Logical Operator/1 -> Switch1/2
  Add4/1 -> Compare To Constant1/1
  Add1/1 -> Compare To Constant/1
  Add3/1 -> Add4/2
  Constant6/1 -> Add4/1
  Add2/1 -> Add1/2
  Constant5/1 -> Add3/2
  Data Store Read3/1 -> Add3/1
  Data Type Conversion/1 -> Mux/1
  Product2/1 -> Data Type Conversion/1
  [SteerK] -> Product2/1
  Switch1/1 -> [SteerK]
  Data Store Read2/1 -> Add2/1
  Constant1/1 -> Add1/1
  Constant3/1 -> Switch1/1
  Constant4/1 -> Add2/2
  Constant2/1 -> Switch1/3
  Mux/1 -> Out1/1
  In1/1 -> Product2/2
  Constant/1 -> Mux/2

== system ZT_VehCtrl_18B/VehCtrl/MontionControl/ValveControl/SteerSys/Subsystem/NATURAL 1 ==
  Action Port : ActionPort
  Constant : Constant  Value=0  OutDataTypeStr=single
  Constant1 : Constant  Value=0  OutDataTypeStr=single
  Mux : Mux  Inputs=2
  Out1 : Outport
  wires:
  Constant1/1 -> Mux/2
  Mux/1 -> Out1/1
  Constant/1 -> Mux/1

== system ZT_VehCtrl_18B/VehCtrl/MontionControl/ValveControl/SteerSys/Subsystem/RIGHT1 ==
  note: 左正右负，右转限制右边幅值
  In1 : Inport
  Action Port : ActionPort
  Add3 : Sum  Inputs=-+
  Add4 : Sum  Inputs=+-
  Add5 : Sum  Inputs=+-
  Add6 : Sum  Inputs=-+
  Compare To Constant : simulink/Logic and Bit Operations/Compare To Constant  relop=>  const=0  OutDataTypeStr=boolean
  Compare To Constant1 : simulink/Logic and Bit Operations/Compare To Constant  relop=>  const=0  OutDataTypeStr=boolean
  Constant1 : Constant
  Constant2 : Constant  Value=0
  Constant4 : Constant  Value=0  OutDataTypeStr=single
  Constant5 : Constant  Value=SteerAngMax
  Constant6 : Constant  Value=steerFLzeroInit
  Constant7 : Constant  Value=steerFRzeroInit
  Constant8 : Constant  Value=SteerAngMax
  Data Store Read1 : DataStoreRead  DataStoreName=SteerAngFR
  Data Store Read2 : DataStoreRead  DataStoreName=SteerAngFL
  Data Type Conversion : DataTypeConversion
  Gain : Gain  Gain=-1
  Gain1 : Gain  Gain=-1
  Logical Operator : Logic  Operator=OR  AllPortsSameDT=off  OutDataTypeStr=boolean
  Mux : Mux  Inputs=2
  Product1 : Product
  Switch1 : Switch  Criteria=u2 > Threshold
  Out1 : Outport
  wires:
  Gain1/1 -> Add6/2
  Gain/1 -> Add3/2
  Add3/1 -> Compare To Constant/1
  Constant8/1 -> Add6/1
  Add4/1 -> Gain/1
  Add5/1 -> Gain1/1
  Add6/1 -> Compare To Constant1/1
  Data Store Read1/1 -> Add5/1
  Compare To Constant/1 -> Logical Operator/1
  Data Store Read2/1 -> Add4/1
  Compare To Constant1/1 -> Logical Operator/2
  Constant5/1 -> Add3/1
  Constant6/1 -> Add4/2
  Constant7/1 -> Add5/2
  Data Type Conversion/1 -> Mux/2
  Product1/1 -> Data Type Conversion/1
  In1/1 -> Product1/1
  [SteerK] -> Product1/2
  Logical Operator/1 -> Switch1/2
  Switch1/1 -> [SteerK]
  Constant2/1 -> Switch1/1
  Constant1/1 -> Switch1/3
  Constant4/1 -> Mux/1
  Mux/1 -> Out1/1
